simulink model "fp_continuous_MIO_16E4"  (R2014a)
settings: Solver=ode5  SolverMode=SingleTasking  StartTime=0.0  StopTime=60  RelTol=1e-3
undefined symbols (not defined in the file): A, B, C, ENCODER_RES, K, L, MIO, MOTOR_SAT, National_Instruments, PCI, TH1_BOUND, TH2_BOUND, TIME_DELAY
libraries: sldrtlib x3
settings Model: SimulationMode=external  CovSFcnEnable=on  ExtModeTrigDuration=60001  Creator=Alunos  LastModifiedBy=samuel
settings OptimizationCC: BlockReduction=off  BooleanDataType=off  SimCompilerOptimization=off
settings DebuggingCC: SaveWithParameterizedLinksMsg=none  UnderspecifiedInitializationDetection=Classic  SignalResolutionControl=TryResolveAllWithWarning  SolverPrmCheckMsg=none  FrameProcessingCompatibilityMsg=error
settings HardwareCC: ProdIntDivRoundTo=Zero  ProdEndianess=LittleEndian  ProdHWDeviceType=Intel->x86/Pentium  TargetIntDivRoundTo=Zero  TargetEndianess=LittleEndian  TargetHWDeviceType=Intel->x86/Pentium
settings RTWCC: SystemTargetFile=rtwin.tlc  TemplateMakefile=rtwin.tmf  Description=Simulink Desktop Real-Time  RTWCompilerOptimization=on
settings CodeAppCC: MaxIdLength=95
settings RTWinTargetCC: TargetPreCompLibLocation=C:\Program Files\MATLAB\R2015a\toolbox\sldrt\lib\win32

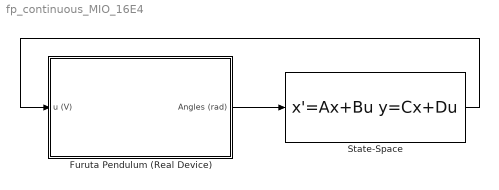
== system fp_continuous_MIO_16E4 ==
  Furuta Pendulum (Real Device) : Subsystem
  State-Space : StateSpace  A=A-B*K-L*C  B=L  C=-K  D=D'  X0=0
  wires:
  Furuta Pendulum (Real Device)/1(Angles (rad)) -> State-Space/1
  State-Space/1 -> Furuta Pendulum (Real Device)/1(u (V))

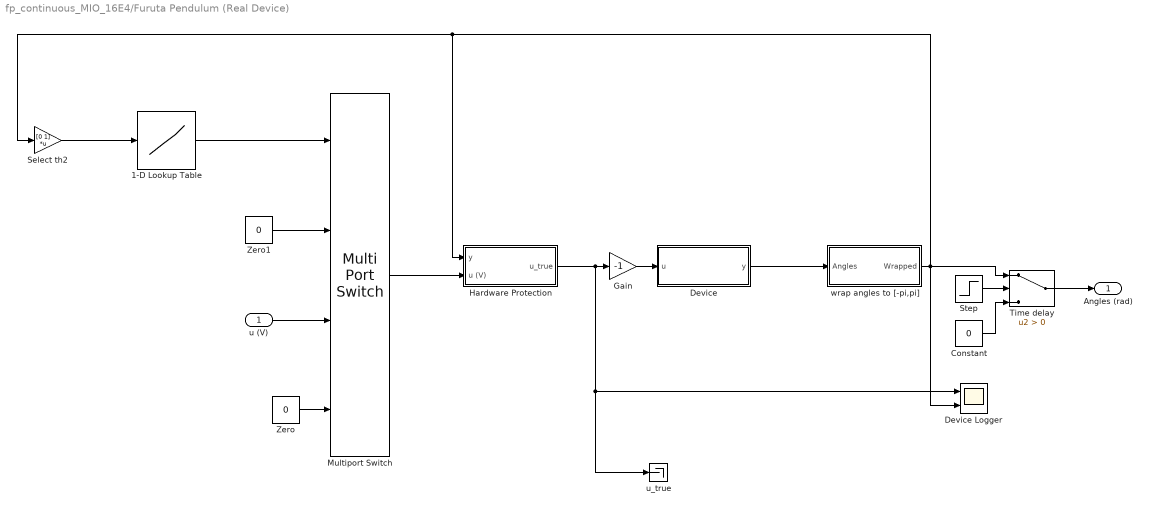
== system fp_continuous_MIO_16E4/Furuta Pendulum (Real Device) ==
  u (V) : Inport
  1-D Lookup Table : Lookup_n-D  NumberOfTableDimensions=1  BreakpointsForDimension1=[-pi,-TH2_BOUND,-TH2_BOUND+.001, 0 TH2_BOUND-.001,TH2_BOUND,pi]  Table=[1 1 2 2 2 1 1]  InternalRulePriority=Speed  RndMeth=Simplest  InputSameDT=on
  Constant : Constant  Value=0
  Device : Subsystem
  Device Logger : Scope  NumInputPorts=2
      settings: YMin=-1~-3.5  YMax=1~3.5  SaveName=DeviceScope  SampleInput=on
  Gain : Gain  Gain=-1
  Hardware Protection : Subsystem
  Multiport Switch : MultiPortSwitch  Inputs=2  DataPortForDefault=Additional data port  DiagnosticForDefault=Warning
  Select th2 : Gain  Gain=[0 1]  Multiplication=Matrix(K*u)
  Step : Step  Time=TIME_DELAY  SampleTime=0
  Time delay : Switch  Criteria=u2 > Threshold
  Zero : Constant  Value=0
  Zero1 : Constant  Value=0
  u_true : Terminator
  wrap angles to [-pi,pi] : Subsystem
  Angles (rad) : Outport
  wires:
  Device/1(y) -> wrap angles to [-pi,pi]/1(Angles)
  wrap angles to [-pi,pi]/1(Wrapped) -> Time delay/1, Device Logger/2, Hardware Protection/1(y), Select th2/1
  Hardware Protection/1(u_true) -> u_true/1, Device Logger/1, Gain/1
  1-D Lookup Table/1 -> Multiport Switch/1
  Multiport Switch/1 -> Hardware Protection/2(u (V))
  Select th2/1 -> 1-D Lookup Table/1
  Zero/1 -> Multiport Switch/4
  Zero1/1 -> Multiport Switch/2
  u (V)/1 -> Multiport Switch/3
  Gain/1 -> Device/1(u)
  Step/1 -> Time delay/2
  Constant/1 -> Time delay/3
  Time delay/1 -> Angles (rad)/1

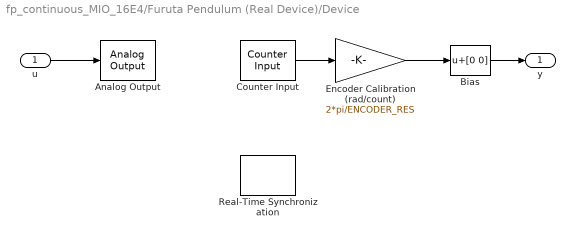
== system fp_continuous_MIO_16E4/Furuta Pendulum (Real Device)/Device ==
  u : Inport
  Analog Output : sldrtlib/Analog Output  SampleTime=0.001  MaxMissedTicks=inf  ShowMissedTicks=off  YieldWhenWaiting=off  DrvName=National_Instruments/PCI-MIO-16E-4  DrvAddress=4294967295  DrvOptions=[0 0 0 0 1 0]  Channels=1  RangeMode=1  VoltRange=1  InitialValue=[]  FinalValue=0
      settings: AttributesFormatString=National Instruments\nPCI-MIO-16E-4 [auto]
  Bias : Bias  Bias=[0 0]
  Counter Input : sldrtlib/Counter Input  SampleTime=0.001  MaxMissedTicks=inf  ShowMissedTicks=off  YieldWhenWaiting=off  DrvName=National_Instruments/PCI-MIO-16E-4  DrvAddress=4294967295  DrvOptions=[0 0 0 0 1 0]  Channels=1:2  ResetMode=1  CounterEdge=1  CounterGate=1  DataType=1
      settings: AttributesFormatString=National Instruments\nPCI-MIO-16E-4 [auto]
  Encoder Calibration (rad/count) : Gain  Gain=2*pi/ENCODER_RES  SaturateOnIntegerOverflow=on  OutDataTypeStr=Inherit: Same as input  ParamDataTypeStr=Inherit: Same as input
  Real-Time Synchronization : sldrtlib/Real-Time Synchronization  SampleTime=0.001  MaxMissedTicks=inf  ShowMissedTicks=off  YieldWhenWaiting=off
  y : Outport
  wires:
  u/1 -> Analog Output/1
  Encoder Calibration (rad/count)/1 -> Bias/1
  Counter Input/1 -> Encoder Calibration (rad/count)/1
  Bias/1 -> y/1

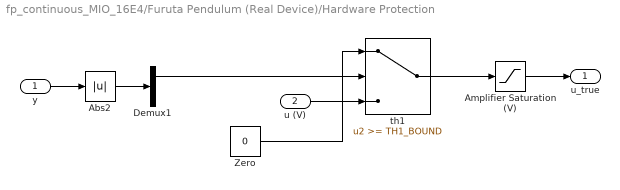
== system fp_continuous_MIO_16E4/Furuta Pendulum (Real Device)/Hardware Protection ==
  y : Inport
  u (V) : Inport  Port=2
  Abs2 : Abs
  Amplifier Saturation (V) : Saturate  UpperLimit=MOTOR_SAT  LowerLimit=-MOTOR_SAT
  Demux1 : Demux  Outputs=2
  Zero : Constant  Value=0
  th1 : Switch  Threshold=TH1_BOUND
  u_true : Outport
  wires:
  Abs2/1 -> Demux1/1
  u (V)/1 -> th1/3
  Zero/1 -> th1/1
  th1/1 -> Amplifier Saturation (V)/1
  Amplifier Saturation (V)/1 -> u_true/1
  y/1 -> Abs2/1
  Demux1/1 -> th1/2

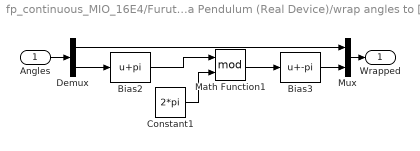
== system fp_continuous_MIO_16E4/Furuta Pendulum (Real Device)/wrap angles to [-pi,pi] ==
  Angles : Inport
  Bias2 : Bias  Bias=pi
  Bias3 : Bias  Bias=-pi
  Constant1 : Constant  Value=2*pi
  Demux : Demux  Outputs=2
  Math Function1 : Math  Operator=mod  SaturateOnIntegerOverflow=on
  Mux : Mux  Inputs=2
  Wrapped : Outport
  wires:
  Bias2/1 -> Math Function1/1
  Constant1/1 -> Math Function1/2
  Math Function1/1 -> Bias3/1
  Angles/1 -> Demux/1
  Demux/2 -> Bias2/1
  Demux/1 -> Mux/1
  Mux/1 -> Wrapped/1
  Bias3/1 -> Mux/2
